simulink model "simulation"  (R2021b)
settings: Solver=VariableStepAuto  StartTime=0.0  StopTime=10.0  RelTol=1e-3
values from neighbouring files (symbols this model uses):
  c0_bar = 1.962390280742725    (= 1.96239028074)    [run_simulation.m]
  DHTABLE = [ pi/2      0         l(1)     q1 ... (first row only)    [compute_vel_obs_gain.m]    (also in dynamic_model_3R_spatial.m = [ pi/2      0      sym('L1') sym('q1'); dynamic_model_simulation.m = [ pi/2      0         l(1)     0; red_obs_gain_computation.m = [ pi/2      0         l(1)     0; run_experiment.m = [ pi/2      0         l(1)     0)
  dq0 = [0.5 -0.5 1]'    [dynamic_model_simulation.m]    (also in run_experiment.m; run_simulation.m = [0., 0., 0.]')
  eta = 1    [compute_vel_obs_gain.m]    (also in dynamic_model_simulation.m; red_obs_gain_computation.m; run_experiment.m; run_simulation.m)
  finite_diff = -1    [run_simulation.m]
  g0 = 9.81    [compute_vel_obs_gain.m]    (also in dynamic_model_3R_spatial.m; dynamic_model_simulation.m; modNE.m = 0; red_obs_gain_computation.m)
  I = zeros(3,3,N)    [compute_vel_obs_gain.m]    (also in dynamic_model_simulation.m; red_obs_gain_computation.m; run_experiment.m; run_simulation.m = zeros(3,3,3))
  K0 = c0bar*(v_max+eta)/(2*lambda_1)    [compute_vel_obs_gain.m]    (also in dynamic_model_simulation.m = 31.0539244645; red_obs_gain_computation.m = 0; run_experiment.m = 103.513081548; run_simulation.m = 62.1078489297)
  K_init = 0.5*dq0'*M*dq0    [run_simulation.m]
  Kd = 3e1    (= 30)    [dynamic_model_simulation.m]    (also in run_experiment.m = 70; run_simulation.m = 50)
  Ko = 5e1    (= 50)    [dynamic_model_simulation.m]    (also in run_experiment.m; run_simulation.m = 10)
  Kp = 3e2    (= 300)    [dynamic_model_simulation.m]    (also in run_experiment.m = 70; run_simulation.m = 100)
  lambda_1 = min(min_first,min_third)/2    [compute_vel_obs_gain.m]    (also in dynamic_model_simulation.m = 0.0947894822263; red_obs_gain_computation.m = min_eig/2; run_experiment.m = 0.0473947411131; run_simulation.m = 0.0473947411131)
  m = [15 10 5]'    [compute_vel_obs_gain.m]    (also in dynamic_model_simulation.m; red_obs_gain_computation.m; run_experiment.m; run_simulation.m = [m1 m2 m3]')
  p_f = [0.,0.8,0.5]    [run_simulation.m]
  p_i = [0.8, 0., 0.5]    [run_simulation.m]
  q0 = inverse_kinematics(p_init,l,soln_type)    [dynamic_model_simulation.m]    (also in run_experiment.m; run_simulation.m = inv_kin(p_i))
  rc = zeros(3,1,3)    [run_simulation.m]
  Timeinterval = [7,9]    [run_simulation.m]
  Timepoints = [0 3 5 7 10]    [run_simulation.m]
  vbar = 2*eta+1    (= 3)    [dynamic_model_simulation.m]    (also in run_simulation.m = 2)
  Velocities = [dq0(1) 2 1 0 -2;dq0(2) 0 2 0 -2;dq0(3) 2 2 0 0]    [run_simulation.m]
  Waypoints = [q0(1) pi/2 pi/4 0 -pi/2; q0(2) pi/4 pi/2 3*pi/4 pi/2; q0(3) pi/2 pi pi/2 -pi/2]    [run_simulation.m]
  x0 = [pi/4,pi/4,1,1,1]'    [compute_vel_obs_gain.m]    (also in dynamic_model_simulation.m = [q0; dq0]; find_c0.m; run_experiment.m = [q0; dq0]; run_simulation.m = [q0;dq0])
  z0 = [0 0 1]'    [dynamic_model_3R_spatial.m]    (also in dynamic_model_simulation.m = x2hat0 - K0*q0; run_experiment.m = x2hat0 - K0*q0; run_simulation.m = x2hat0-K0*q0)
undefined symbols (not defined in the file or in its folder): eul2tform, trvec2tform
libraries: robotcorelib x5, simulink x2, robotmaniplib x1
settings Model: Creator=lyuk  LastModifiedBy=lyuk

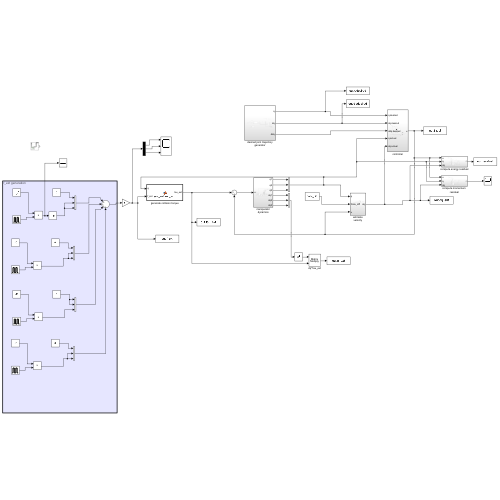
[thumbnail: Simulink's stored preview of the top-level diagram]
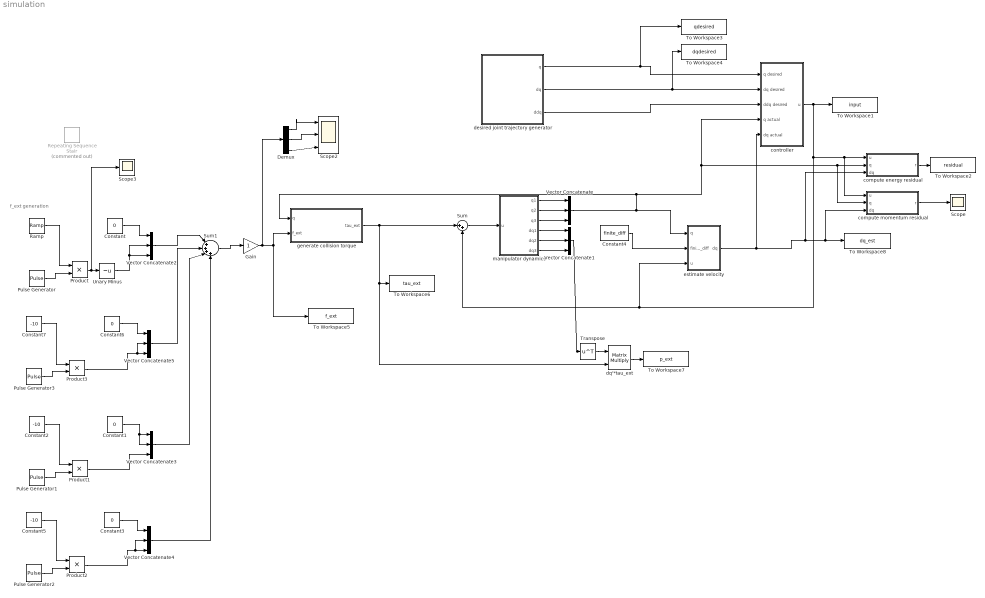
== system simulation ==
  note: f_ext generation
  Constant{,1,3,6} (4 alike) : Constant  Value=0
  Constant2 : Constant  Value=-10
  Constant4 : Constant  Value=finite_diff
  Constant5 : Constant  Value=-10
  Constant7 : Constant  Value=-10
  Demux : Demux  Outputs=3
  Gain : Gain
  Product{,1..3} (4 alike) : Product
  Pulse Generator : DiscretePulseGenerator  PulseType=Time based  Period=10  PulseWidth=20  PhaseDelay=1
  Pulse Generator1 : DiscretePulseGenerator  PulseType=Time based  Period=10  PulseWidth=5  PhaseDelay=7.5
  Pulse Generator2 : DiscretePulseGenerator  PulseType=Time based  Period=10  PulseWidth=5  PhaseDelay=8.5
  Pulse Generator3 : DiscretePulseGenerator  PulseType=Time based  Period=10  PulseWidth=5  PhaseDelay=5
  Ramp : simulink/Sources/Ramp  slope=8  start=1  InitialOutput=0
  Repeating Sequence Stair : simulink/Sources/Repeating Sequence Stair  Commented=on  OutValues=[3 5 15].'  tsamp=-1  OutMin=[]  OutMax=[]  OutDataTypeStr=double  OutputDataTypeScalingMode=double  OutDataType=fixdt(0,8)  ConRadixGroup=Best Precision: Vector-wise  OutScaling=2^-12
  Scope : Scope
  Scope2 : Scope  NumInputPorts=3
  Scope3 : Scope
  Sum : Sum  Inputs=|++
  Sum1 : Sum  Inputs=|++++
  To Workspace1 : ToWorkspace  VariableName=input  SampleTime=-1
  To Workspace2 : ToWorkspace  VariableName=residual  SampleTime=-1
      settings: Save2DSignal=2-D array (concatenate along first dimension)
  To Workspace3 : ToWorkspace  VariableName=qdesired  SampleTime=-1
  To Workspace4 : ToWorkspace  VariableName=dqdesired  SampleTime=-1
  To Workspace5 : ToWorkspace  VariableName=f_ext  SampleTime=-1
  To Workspace6 : ToWorkspace  VariableName=tau_ext  SampleTime=-1
  To Workspace7 : ToWorkspace  VariableName=p_ext  SampleTime=-1
      settings: Save2DSignal=2-D array (concatenate along first dimension)
  To Workspace8 : ToWorkspace  VariableName=dq_est  SampleTime=-1
  Transpose : Math  Operator=transpose  SaturateOnIntegerOverflow=on
  Unary Minus : UnaryMinus
  Vector Concatenate{,1..5} (6 alike) : Concatenate  NumInputs=3  Mode=Multidimensional array
  compute energy residual : Subsystem
  compute momentum residual : Subsystem
  controller : Subsystem
  desired joint trajectory generator : Subsystem
  dq'*tau_ext : Product  Multiplication=Matrix(*)
  estimate velocity : Subsystem
  generate collision torque : MATLAB Function  TreatAsAtomicUnit=on
  manipulator dynamics : Subsystem
  wires:
  manipulator dynamics/2(q2) -> Vector Concatenate/2
  manipulator dynamics/3(q3) -> Vector Concatenate/3
  manipulator dynamics/1(q1) -> Vector Concatenate/1
  manipulator dynamics/4(dq1) -> Vector Concatenate1/1
  manipulator dynamics/5(dq2) -> Vector Concatenate1/2
  manipulator dynamics/6(dq3) -> Vector Concatenate1/3
  Vector Concatenate1/1 -> Transpose/1
  controller/1(u) -> To Workspace1/1, compute momentum residual/1(u), compute energy residual/1(u), estimate velocity/3(u), Sum/2
  compute energy residual/1(r) -> To Workspace2/1
  generate collision torque/1(tau_ext) -> To Workspace6/1, dq'*tau_ext/2, Sum/1
  Sum/1 -> manipulator dynamics/1(u)
  Transpose/1 -> dq'*tau_ext/1
  dq'*tau_ext/1 -> To Workspace7/1
  Product/1 -> Scope3/1, Unary Minus/1
  Pulse Generator/1 -> Product/2
  Ramp/1 -> Product/1
  Vector Concatenate/1 -> estimate velocity/1(q), compute momentum residual/2(q), compute energy residual/2(q), controller/4(q actual), generate collision torque/1(q)
  Unary Minus/1 -> Vector Concatenate2/2, Vector Concatenate2/3
  Constant/1 -> Vector Concatenate2/1
  Gain/1 -> Demux/1, To Workspace5/1, generate collision torque/2(f_ext)
  estimate velocity/1(dq) -> controller/5(dq actual), compute energy residual/3(dq), compute momentum residual/3(dq), To Workspace8/1
  Constant4/1 -> estimate velocity/2(finite_diff)
  compute momentum residual/1(r) -> Scope/1
  desired joint trajectory generator/1(q) -> To Workspace3/1, controller/1(q desired)
  desired joint trajectory generator/2(dq) -> To Workspace4/1, controller/2(dq desired)
  desired joint trajectory generator/3(ddq) -> controller/3(ddq desired)
  Constant1/1 -> Vector Concatenate3/2, Vector Concatenate3/1
  Product1/1 -> Vector Concatenate3/3
  Constant2/1 -> Product1/1
  Pulse Generator1/1 -> Product1/2
  Sum1/1 -> Gain/1
  Vector Concatenate2/1 -> Sum1/1
  Pulse Generator2/1 -> Product2/2
  Constant5/1 -> Product2/1
  Product2/1 -> Vector Concatenate4/2, Vector Concatenate4/3
  Constant3/1 -> Vector Concatenate4/1
  Pulse Generator3/1 -> Product3/2
  Constant7/1 -> Product3/1
  Product3/1 -> Vector Concatenate5/2, Vector Concatenate5/3
  Constant6/1 -> Vector Concatenate5/1
  Vector Concatenate5/1 -> Sum1/2
  Vector Concatenate3/1 -> Sum1/3
  Vector Concatenate4/1 -> Sum1/4
  Demux/1 -> Scope2/1
  Demux/2 -> Scope2/2
  Demux/3 -> Scope2/3

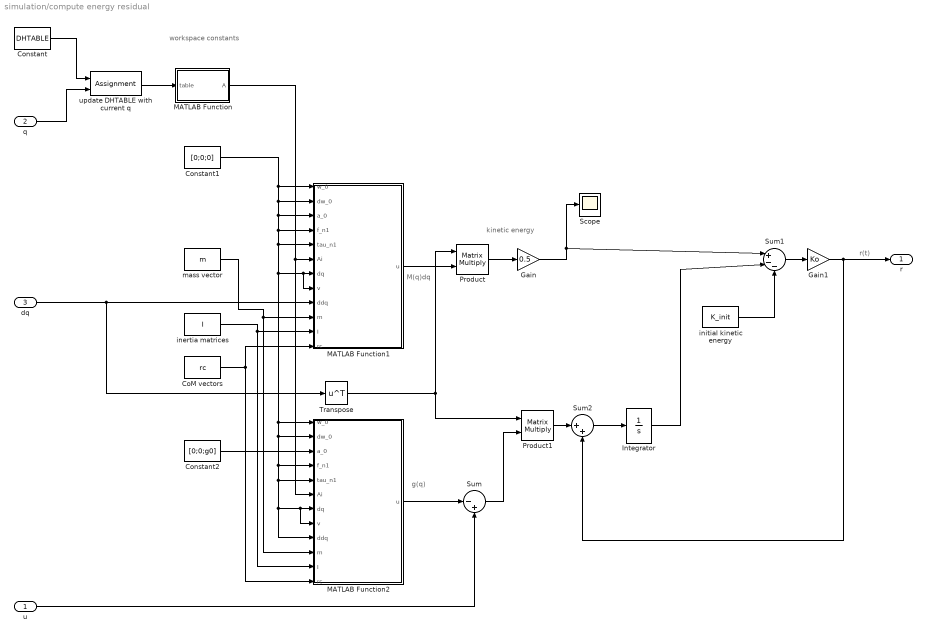
== system simulation/compute energy residual ==
  note: r(t)
  note: g(q)
  note: kinetic energy
  note: M(q)dq
  note: workspace constants
  u : Inport
  q : Inport  Port=2
  dq : Inport  Port=3
  CoM vectors : Constant  Value=rc  VectorParams1D=off
  Constant : Constant  Value=DHTABLE  VectorParams1D=off
  Constant1 : Constant  Value=[0;0;0]  VectorParams1D=off
  Constant2 : Constant  Value=[0;0;g0]  VectorParams1D=off
  Gain : Gain  Gain=0.5
  Gain1 : Gain  Gain=Ko
  Integrator : Integrator
  MATLAB Function : MATLAB Function  TreatAsAtomicUnit=on
  MATLAB Function1 : MATLAB Function  TreatAsAtomicUnit=on
  MATLAB Function2 : MATLAB Function  TreatAsAtomicUnit=on
  Product : Product  Multiplication=Matrix(*)
  Product1 : Product  Multiplication=Matrix(*)
  Scope : Scope
  Sum : Sum  Inputs=|-+
  Sum1 : Sum  Inputs=|+--
  Sum2 : Sum  Inputs=|++
  Transpose : Math  Operator=transpose  SaturateOnIntegerOverflow=on
  inertia matrices : Constant  Value=I  VectorParams1D=off
  initial kinetic energy : Constant  Value=K_init  VectorParams1D=off
  mass vector : Constant  Value=m  VectorParams1D=off
  update DHTABLE with current q : Assignment  NumberOfDimensions=2  DiagnosticForDimensions=Warning  IndexOptions=Assign all,Index vector (dialog)  Indices=1,[4]  OutputSizes=1,1
  r : Outport
  wires:
  mass vector/1 -> MATLAB Function1/10(m), MATLAB Function2/10(m)
  inertia matrices/1 -> MATLAB Function1/11(I), MATLAB Function2/11(I)
  Constant1/1 -> MATLAB Function2/9(ddq), MATLAB Function2/8(v), MATLAB Function2/7(dq), MATLAB Function2/5(tau_n1), MATLAB Function2/4(f_n1), MATLAB Function2/2(dw_0), MATLAB Function2/1(w_0), MATLAB Function1/8(v), MATLAB Function1/7(dq), MATLAB Function1/5(tau_n1), MATLAB Function1/4(f_n1), MATLAB Function1/3(a_0), MATLAB Function1/2(dw_0), MATLAB Function1/1(w_0)
  CoM vectors/1 -> MATLAB Function1/12(rc), MATLAB Function2/12(rc)
  update DHTABLE with current q/1 -> MATLAB Function/1(table)
  Constant/1 -> update DHTABLE with current q/1
  MATLAB Function/1(A) -> MATLAB Function2/6(Ai), MATLAB Function1/6(Ai)
  q/1 -> update DHTABLE with current q/2
  dq/1 -> Transpose/1, MATLAB Function1/9(ddq)
  MATLAB Function1/1(u) -> Product/2
  Transpose/1 -> Product/1, Product1/1
  Product/1 -> Gain/1
  Constant2/1 -> MATLAB Function2/3(a_0)
  Gain1/1 -> Sum2/2, r/1
  u/1 -> Sum/2
  Sum/1 -> Product1/2
  Gain/1 -> Scope/1, Sum1/1
  Integrator/1 -> Sum1/2
  Sum1/1 -> Gain1/1
  Product1/1 -> Sum2/1
  Sum2/1 -> Integrator/1
  MATLAB Function2/1(u) -> Sum/1
  initial kinetic energy/1 -> Sum1/3

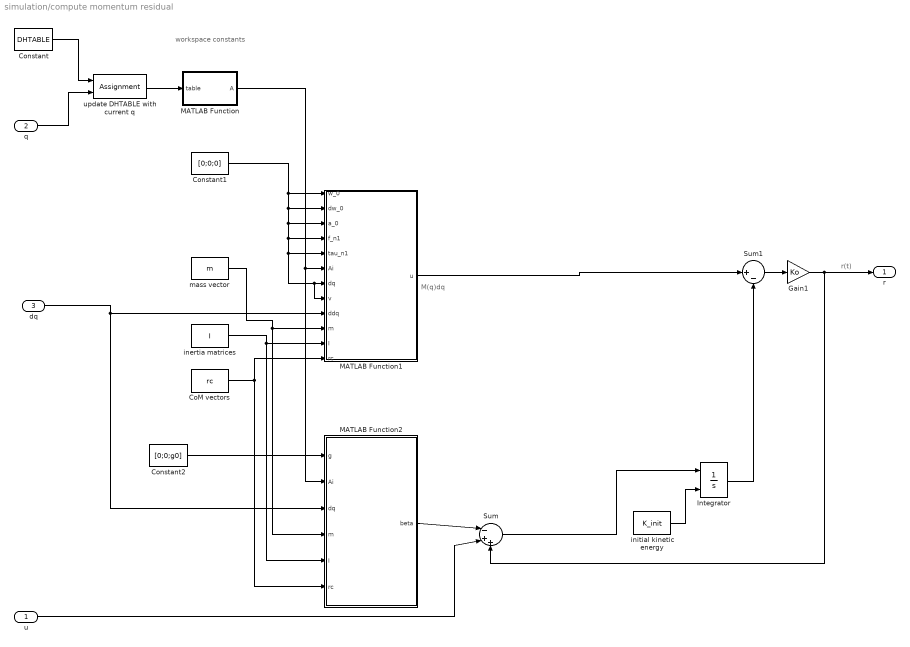
== system simulation/compute momentum residual ==
  note: workspace constants
  note: M(q)dq
  note: r(t)
  u : Inport
  q : Inport  Port=2
  dq : Inport  Port=3
  CoM vectors : Constant  Value=rc  VectorParams1D=off
  Constant : Constant  Value=DHTABLE  VectorParams1D=off
  Constant1 : Constant  Value=[0;0;0]  VectorParams1D=off
  Constant2 : Constant  Value=[0;0;g0]  VectorParams1D=off
  Gain1 : Gain  Gain=Ko
  Integrator : Integrator  InitialConditionSource=external
  MATLAB Function : MATLAB Function  TreatAsAtomicUnit=on
  MATLAB Function1 : MATLAB Function  TreatAsAtomicUnit=on
  MATLAB Function2 : MATLAB Function  TreatAsAtomicUnit=on
  Sum : Sum  Inputs=|-++
  Sum1 : Sum  Inputs=|+-
  inertia matrices : Constant  Value=I  VectorParams1D=off
  initial kinetic energy : Constant  Value=K_init  VectorParams1D=off
  mass vector : Constant  Value=m  VectorParams1D=off
  update DHTABLE with current q : Assignment  NumberOfDimensions=2  DiagnosticForDimensions=Warning  IndexOptions=Assign all,Index vector (dialog)  Indices=1,[4]  OutputSizes=1,1
  r : Outport
  wires:
  Sum/1 -> Integrator/1
  initial kinetic energy/1 -> Integrator/2
  Sum1/1 -> Gain1/1
  Integrator/1 -> Sum1/2
  u/1 -> Sum/2
  MATLAB Function2/1(beta) -> Sum/1
  Gain1/1 -> Sum/3, r/1
  Constant2/1 -> MATLAB Function2/1(g)
  MATLAB Function1/1(u) -> Sum1/1
  dq/1 -> MATLAB Function1/9(ddq), MATLAB Function2/3(dq)
  q/1 -> update DHTABLE with current q/2
  MATLAB Function/1(A) -> MATLAB Function1/6(Ai), MATLAB Function2/2(Ai)
  Constant/1 -> update DHTABLE with current q/1
  update DHTABLE with current q/1 -> MATLAB Function/1(table)
  CoM vectors/1 -> MATLAB Function2/6(rc), MATLAB Function1/12(rc)
  Constant1/1 -> MATLAB Function1/1(w_0), MATLAB Function1/2(dw_0), MATLAB Function1/3(a_0), MATLAB Function1/4(f_n1), MATLAB Function1/5(tau_n1), MATLAB Function1/7(dq), MATLAB Function1/8(v)
  inertia matrices/1 -> MATLAB Function2/5(I), MATLAB Function1/11(I)
  mass vector/1 -> MATLAB Function2/4(m), MATLAB Function1/10(m)

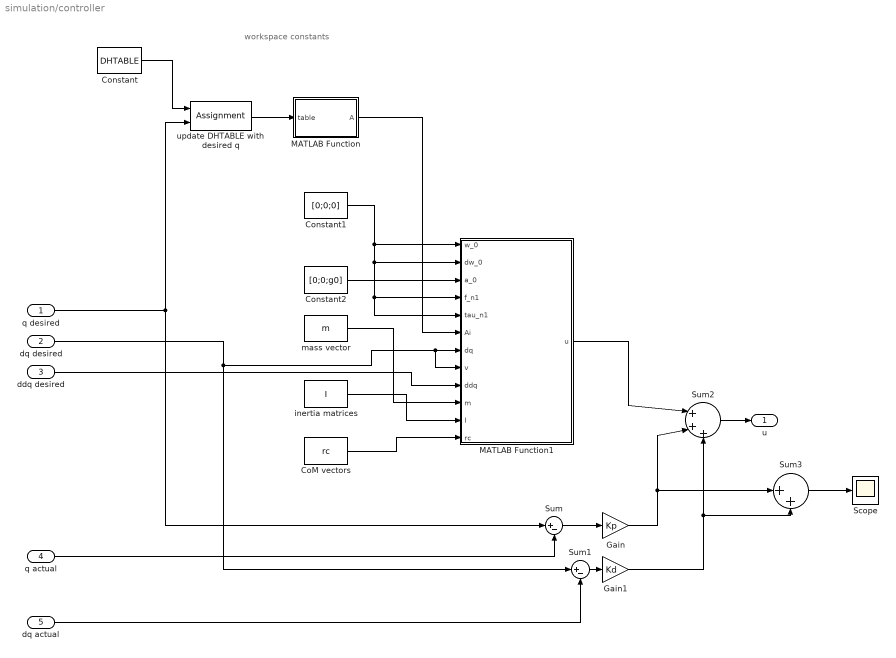
== system simulation/controller ==
  note: workspace constants
  q desired : Inport
  dq desired : Inport  Port=2
  ddq desired : Inport  Port=3
  q actual : Inport  Port=4
  dq actual : Inport  Port=5
  CoM vectors : Constant  Value=rc  VectorParams1D=off
  Constant : Constant  Value=DHTABLE  VectorParams1D=off
  Constant1 : Constant  Value=[0;0;0]  VectorParams1D=off
  Constant2 : Constant  Value=[0;0;g0]  VectorParams1D=off
  Gain : Gain  Gain=Kp
  Gain1 : Gain  Gain=Kd
  MATLAB Function : MATLAB Function  TreatAsAtomicUnit=on
  MATLAB Function1 : MATLAB Function  TreatAsAtomicUnit=on
  Scope : Scope
  Sum : Sum  Inputs=|+-
  Sum1 : Sum  Inputs=|+-
  Sum2 : Sum  Inputs=|+++
  Sum3 : Sum  Inputs=|++
  inertia matrices : Constant  Value=I  VectorParams1D=off
  mass vector : Constant  Value=m  VectorParams1D=off
  update DHTABLE with desired q : Assignment  NumberOfDimensions=2  DiagnosticForDimensions=Warning  IndexOptions=Assign all,Index vector (dialog)  Indices=1,[4]  OutputSizes=1,1
  u : Outport
  wires:
  Gain1/1 -> Sum3/2, Sum2/3
  update DHTABLE with desired q/1 -> MATLAB Function/1(table)
  Gain/1 -> Sum2/2, Sum3/1
  Constant/1 -> update DHTABLE with desired q/1
  Constant1/1 -> MATLAB Function1/2(dw_0), MATLAB Function1/5(tau_n1), MATLAB Function1/4(f_n1), MATLAB Function1/1(w_0)
  inertia matrices/1 -> MATLAB Function1/11(I)
  CoM vectors/1 -> MATLAB Function1/12(rc)
  Constant2/1 -> MATLAB Function1/3(a_0)
  mass vector/1 -> MATLAB Function1/10(m)
  MATLAB Function/1(A) -> MATLAB Function1/6(Ai)
  Sum1/1 -> Gain1/1
  q desired/1 -> Sum/1, update DHTABLE with desired q/2
  dq desired/1 -> MATLAB Function1/8(v), MATLAB Function1/7(dq), Sum1/1
  ddq desired/1 -> MATLAB Function1/9(ddq)
  dq actual/1 -> Sum1/2
  Sum/1 -> Gain/1
  q actual/1 -> Sum/2
  Sum3/1 -> Scope/1
  Sum2/1 -> u/1
  MATLAB Function1/1(u) -> Sum2/1

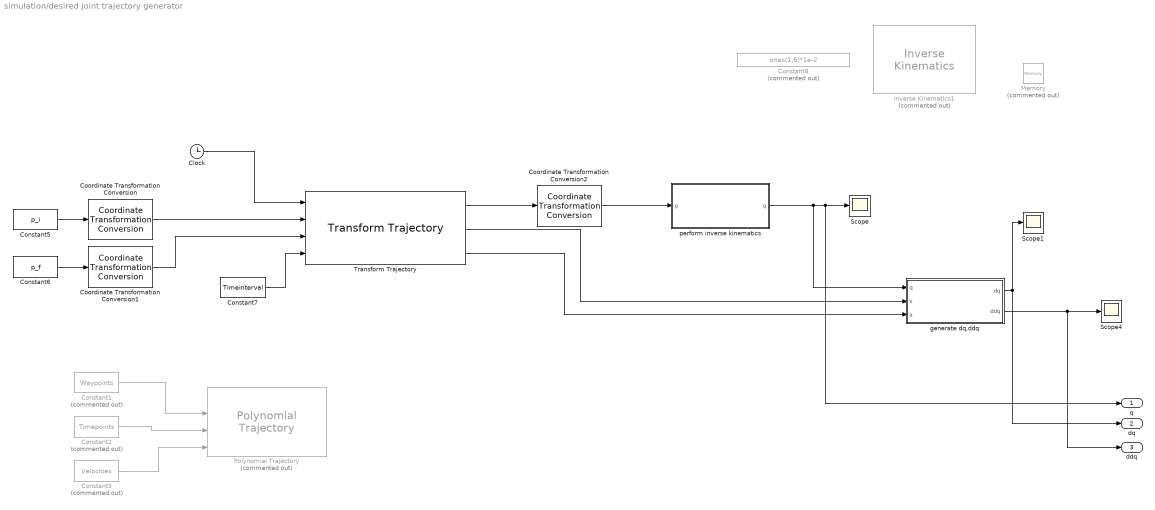
== system simulation/desired joint trajectory generator ==
  Clock : Clock
  Constant1 : Constant  Commented=on  Value=Waypoints
  Constant2 : Constant  Commented=on  Value=Timepoints
  Constant3 : Constant  Commented=on  Value=Velocities
  Constant5 : Constant  Value=p_i
  Constant6 : Constant  Value=p_f
  Constant7 : Constant  Value=Timeinterval
  Constant8 : Constant  Commented=on  Value=ones(1,6)*1e-2
  Coordinate Transformation Conversion : robotcorelib/Coordinate Transformation Conversion  InputRepresentation=Translation Vector  InputEulerSequence=ZYX  ShowTrVecInputPort=on  OutputRepresentation=Homogeneous Transformation  OutputEulerSequence=ZYX  ShowTrVecOutputPort=on  SimulateUsing=Interpreted execution
      settings: SourceProductBaseCode=NV,RO,RR,UV
  Coordinate Transformation Conversion1 : robotcorelib/Coordinate Transformation Conversion  InputRepresentation=Translation Vector  InputEulerSequence=ZYX  ShowTrVecInputPort=on  OutputRepresentation=Homogeneous Transformation  OutputEulerSequence=ZYX  ShowTrVecOutputPort=on  SimulateUsing=Interpreted execution
      settings: SourceProductBaseCode=NV,RO,RR,UV
  Coordinate Transformation Conversion2 : robotcorelib/Coordinate Transformation Conversion  InputRepresentation=Homogeneous Transformation  InputEulerSequence=ZYX  ShowTrVecInputPort=on  OutputRepresentation=Translation Vector  OutputEulerSequence=ZYX  ShowTrVecOutputPort=on  SimulateUsing=Interpreted execution
      settings: SourceProductBaseCode=NV,RO,RR,UV
  Inverse Kinematics1 : robotmaniplib/Inverse Kinematics  Commented=on  RigidBodyTree=robot  EndEffector=body3  ShowInfo=on  SolverName=BFGS Gradient Projection  EnforceJointLimits=on  MaxIterations=1500  MaxTime=10  GradientTolerance=1e-7  SolutionTolerance=1e-6  StepTolerance=1e-14  ErrorChangeTolerance=1e-12  UseErrorDamping=on  DampingBias=0.0025  SimulateUsing=Interpreted execution
  Memory : Memory  Commented=on  InitialCondition=q0  InheritSampleTime=on
  Polynomial Trajectory : robotcorelib/Polynomial Trajectory  Commented=on  WaypointSource=External  Waypoints=[q0(1) pi/2 pi; q0(2) pi/4 pi/2; q0(3) pi/2 0]  TimePoints=[0 5 10 ]  TimeInterval=[ 1, 4 ]  Method=Cubic Polynomial  ParameterSource=External  VelocityBoundaryCondition=[dq0(1) zeros(1,2);dq0(2) zeros(1,2);dq0(3) zeros(1,2)]  AccelerationBoundaryCondition=zeros( 2, 5 )  SimulateUsing=Interpreted execution
  Scope : Scope
  Scope1 : Scope
  Scope4 : Scope
  Transform Trajectory : robotcorelib/Transform Trajectory  WaypointSource=External  T0=trvec2tform( [ 1, 10, -1 ] )  TF=eul2tform( [ 0, pi, pi / 2 ] )  TimeInterval=[ 2, 3 ]  CustomTimeScaling=off  ParameterSource=Internal  TSTime=2:0.1:3  TimeScaling=[ 0:0.1:1; ones( 1, 11 ); zeros( 1, 11 ) ]  SimulateUsing=Interpreted execution
      settings: SourceProductBaseCode=NV,RO,RR,UV
  generate dq,ddq : MATLAB Function  TreatAsAtomicUnit=on
  perform inverse kinematics : MATLAB Function  TreatAsAtomicUnit=on
  q : Outport
  dq : Outport  Port=2
  ddq : Outport  Port=3
  wires:
  perform inverse kinematics/1(q) -> q/1, Scope/1, generate dq,ddq/1(q)
  Constant2/1 -> Polynomial Trajectory/3
  Constant3/1 -> Polynomial Trajectory/4
  Clock/1 -> Transform Trajectory/1
  Constant1/1 -> Polynomial Trajectory/2
  Constant7/1 -> Transform Trajectory/4
  Transform Trajectory/2 -> generate dq,ddq/2(v)
  Transform Trajectory/3 -> generate dq,ddq/3(a)
  generate dq,ddq/1(dq) -> dq/1, Scope1/1
  generate dq,ddq/2(ddq) -> Scope4/1, ddq/1
  Constant5/1 -> Coordinate Transformation Conversion/1
  Coordinate Transformation Conversion/1 -> Transform Trajectory/2
  Constant6/1 -> Coordinate Transformation Conversion1/1
  Coordinate Transformation Conversion1/1 -> Transform Trajectory/3
  Coordinate Transformation Conversion2/1 -> perform inverse kinematics/1(p)
  Transform Trajectory/1 -> Coordinate Transformation Conversion2/1

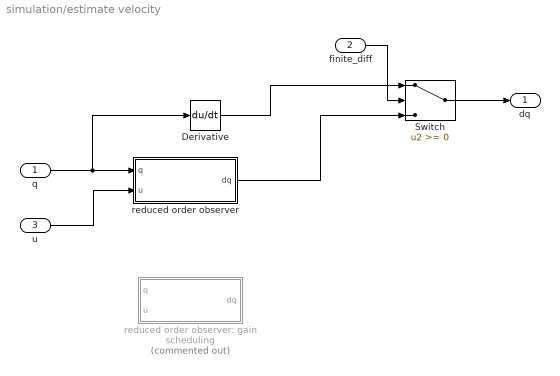
== system simulation/estimate velocity ==
  q : Inport
  finite_diff : Inport  Port=2
  u : Inport  Port=3
  Derivative : Derivative
  Switch : Switch
  reduced order observer : Subsystem
  reduced order observer: gain scheduling : Subsystem  Commented=on
  dq : Outport
  wires:
  q/1 -> Derivative/1, reduced order observer/1(q)
  reduced order observer/1(dq) -> Switch/3
  Switch/1 -> dq/1
  Derivative/1 -> Switch/1
  finite_diff/1 -> Switch/2
  u/1 -> reduced order observer/2(u)

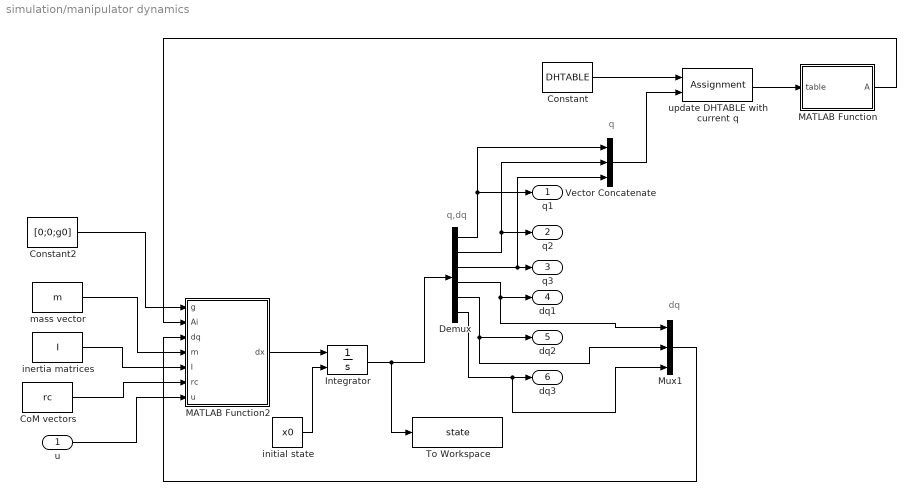
== system simulation/manipulator dynamics ==
  note: q
  note: q,dq
  note: dq
  u : Inport
  CoM vectors : Constant  Value=rc  VectorParams1D=off
  Constant : Constant  Value=DHTABLE  VectorParams1D=off
  Constant2 : Constant  Value=[0;0;g0]  VectorParams1D=off
  Demux : Demux  Outputs=6
  Integrator : Integrator  InitialConditionSource=external  InitialCondition=[q0;dq0]
  MATLAB Function : MATLAB Function  TreatAsAtomicUnit=on
  MATLAB Function2 : MATLAB Function  TreatAsAtomicUnit=on
  Mux1 : Mux  Inputs=3
  To Workspace : ToWorkspace  VariableName=state  SampleTime=-1
  Vector Concatenate : Concatenate  NumInputs=3  Mode=Multidimensional array
  inertia matrices : Constant  Value=I  VectorParams1D=off
  initial state : Constant  Value=x0  VectorParams1D=off
  mass vector : Constant  Value=m  VectorParams1D=off
  update DHTABLE with current q : Assignment  NumberOfDimensions=2  DiagnosticForDimensions=Warning  IndexOptions=Assign all,Index vector (dialog)  Indices=1,[4]  OutputSizes=1,1
  q1 : Outport
  q2 : Outport  Port=2
  q3 : Outport  Port=3
  dq1 : Outport  Port=4
  dq2 : Outport  Port=5
  dq3 : Outport  Port=6
  wires:
  Demux/1 -> q1/1, Vector Concatenate/1
  Integrator/1 -> To Workspace/1, Demux/1
  Demux/6 -> Mux1/3, dq3/1
  Demux/4 -> Mux1/1, dq1/1
  u/1 -> MATLAB Function2/7(u)
  Demux/2 -> Vector Concatenate/2, q2/1
  MATLAB Function2/1(dx) -> Integrator/1
  Demux/3 -> Vector Concatenate/3, q3/1
  Demux/5 -> dq2/1, Mux1/2
  update DHTABLE with current q/1 -> MATLAB Function/1(table)
  mass vector/1 -> MATLAB Function2/4(m)
  inertia matrices/1 -> MATLAB Function2/5(I)
  CoM vectors/1 -> MATLAB Function2/6(rc)
  Mux1/1 -> MATLAB Function2/3(dq)
  Vector Concatenate/1 -> update DHTABLE with current q/2
  Constant/1 -> update DHTABLE with current q/1
  MATLAB Function/1(A) -> MATLAB Function2/2(Ai)
  Constant2/1 -> MATLAB Function2/1(g)
  initial state/1 -> Integrator/2

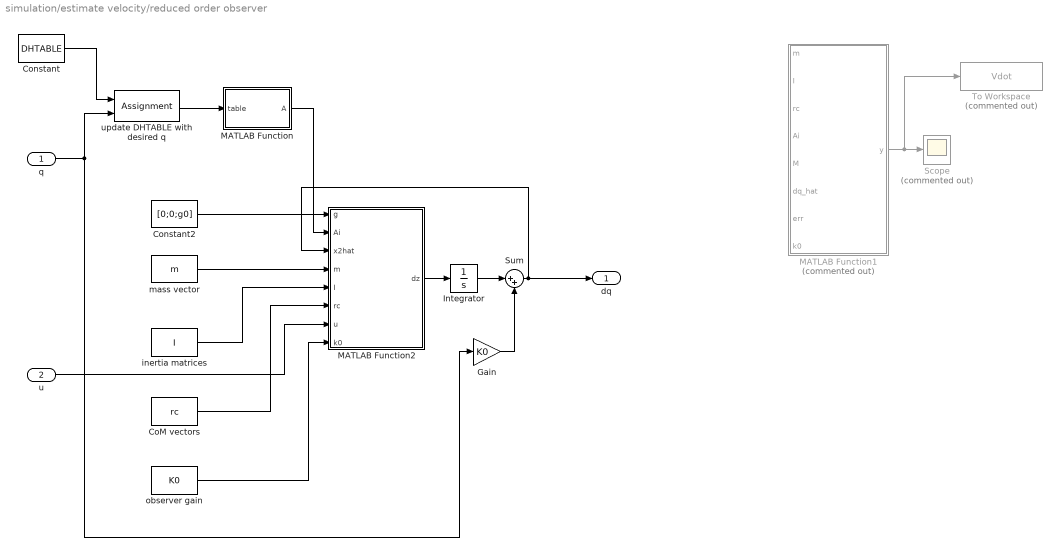
== system simulation/estimate velocity/reduced order observer ==
  q : Inport
  u : Inport  Port=2
  CoM vectors : Constant  Value=rc  VectorParams1D=off
  Constant : Constant  Value=DHTABLE  VectorParams1D=off
  Constant2 : Constant  Value=[0;0;g0]  VectorParams1D=off
  Gain : Gain  Gain=K0
  Integrator : Integrator  InitialCondition=z0
  MATLAB Function : MATLAB Function  TreatAsAtomicUnit=on
  MATLAB Function1 : MATLAB Function  Commented=on  TreatAsAtomicUnit=on
  MATLAB Function2 : MATLAB Function  TreatAsAtomicUnit=on
  Scope : Scope  Commented=on
  Sum : Sum  Inputs=|++
  To Workspace : ToWorkspace  Commented=on  VariableName=Vdot  SampleTime=-1
  inertia matrices : Constant  Value=I  VectorParams1D=off
  mass vector : Constant  Value=m  VectorParams1D=off
  observer gain : Constant  Value=K0  VectorParams1D=off
  update DHTABLE with desired q : Assignment  NumberOfDimensions=2  DiagnosticForDimensions=Warning  IndexOptions=Assign all,Index vector (dialog)  Indices=1,[4]  OutputSizes=1,1
  dq : Outport
  wires:
  CoM vectors/1 -> MATLAB Function2/6(rc)
  inertia matrices/1 -> MATLAB Function2/5(I)
  mass vector/1 -> MATLAB Function2/4(m)
  Constant2/1 -> MATLAB Function2/1(g)
  update DHTABLE with desired q/1 -> MATLAB Function/1(table)
  Constant/1 -> update DHTABLE with desired q/1
  q/1 -> update DHTABLE with desired q/2, Gain/1
  MATLAB Function/1(A) -> MATLAB Function2/2(Ai)
  observer gain/1 -> MATLAB Function2/8(k0)
  u/1 -> MATLAB Function2/7(u)
  MATLAB Function2/1(dz) -> Integrator/1
  Integrator/1 -> Sum/1
  Gain/1 -> Sum/2
  Sum/1 -> dq/1, MATLAB Function2/3(x2hat)
  MATLAB Function1/1(y) -> To Workspace/1, Scope/1

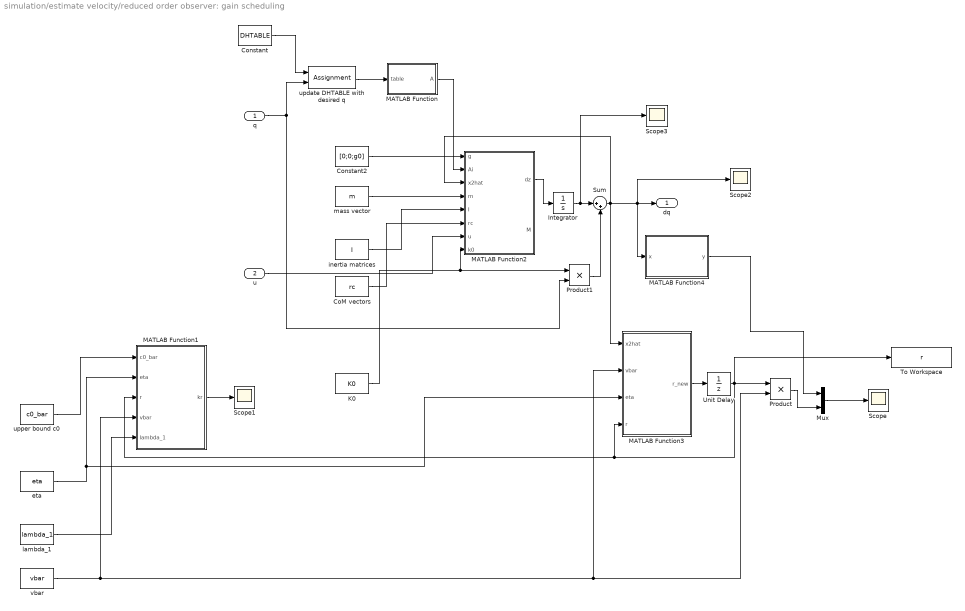
== system simulation/estimate velocity/reduced order observer: gain scheduling ==
  q : Inport
  u : Inport  Port=2
  CoM vectors : Constant  Value=rc  VectorParams1D=off
  Constant : Constant  Value=DHTABLE  VectorParams1D=off
  Constant2 : Constant  Value=[0;0;g0]  VectorParams1D=off
  Integrator : Integrator  InitialCondition=z0
  K0 : Constant  Value=K0  VectorParams1D=off
  MATLAB Function : MATLAB Function  TreatAsAtomicUnit=on
  MATLAB Function1 : MATLAB Function  TreatAsAtomicUnit=on
  MATLAB Function2 : MATLAB Function  TreatAsAtomicUnit=on
  MATLAB Function3 : MATLAB Function  TreatAsAtomicUnit=on
  MATLAB Function4 : MATLAB Function  TreatAsAtomicUnit=on
  Mux : Mux  Inputs=2
  Product : Product
  Product1 : Product
  Scope{,1..3} (4 alike) : Scope
  Sum : Sum  Inputs=|++
  To Workspace : ToWorkspace  VariableName=r  SaveFormat=Structure With Time  SampleTime=-1
  Unit Delay : UnitDelay  InitialCondition=1  SampleTime=-1  HasFrameUpgradeWarning=on
  eta : Constant  Value=eta  VectorParams1D=off
  inertia matrices : Constant  Value=I  VectorParams1D=off
  lambda_1 : Constant  Value=lambda_1  VectorParams1D=off
  mass vector : Constant  Value=m  VectorParams1D=off
  update DHTABLE with desired q : Assignment  NumberOfDimensions=2  DiagnosticForDimensions=Warning  IndexOptions=Assign all,Index vector (dialog)  Indices=1,[4]  OutputSizes=1,1
  upper bound c0 : Constant  Value=c0_bar  VectorParams1D=off
  vbar : Constant  Value=vbar  VectorParams1D=off
  dq : Outport
  wires:
  Sum/1 -> Scope2/1, MATLAB Function4/1(x), dq/1, MATLAB Function3/1(x2hat), MATLAB Function2/3(x2hat)
  Product1/1 -> Sum/2
  Integrator/1 -> Scope3/1, Sum/1
  MATLAB Function2/1(dz) -> Integrator/1
  u/1 -> MATLAB Function2/7(u)
  MATLAB Function/1(A) -> MATLAB Function2/2(Ai)
  q/1 -> Product1/2, update DHTABLE with desired q/2
  Constant/1 -> update DHTABLE with desired q/1
  update DHTABLE with desired q/1 -> MATLAB Function/1(table)
  Constant2/1 -> MATLAB Function2/1(g)
  mass vector/1 -> MATLAB Function2/4(m)
  inertia matrices/1 -> MATLAB Function2/5(I)
  CoM vectors/1 -> MATLAB Function2/6(rc)
  upper bound c0/1 -> MATLAB Function1/1(c0_bar)
  eta/1 -> MATLAB Function3/3(eta), MATLAB Function1/2(eta)
  lambda_1/1 -> MATLAB Function1/5(lambda_1)
  vbar/1 -> MATLAB Function1/4(vbar), Product/2, MATLAB Function3/2(vbar)
  MATLAB Function3/1(r_new) -> Unit Delay/1
  MATLAB Function1/1(kr) -> Scope1/1
  MATLAB Function4/1(y) -> Mux/1
  Product/1 -> Mux/2
  Mux/1 -> Scope/1
  Unit Delay/1 -> MATLAB Function3/4(r), MATLAB Function1/3(r), To Workspace/1, Product/1
  K0/1 -> MATLAB Function2/8(k0), Product1/1

== matlab function simulation/compute momentum residual/MATLAB Function ==
  data: table input; A output
function A = DHMatrix(table)
% inputs:
%  -table: the DH parameters table, a n-vector of vectors composed with 
%  this structure: [alpha a d theta]
% output:
%  -A: cell array with homogeneous relative transformations from RF i-1 to
%   RF i
    nums = size(table);
    
    A = zeros(4,4,nums(1));
    
    for i = 1:nums(1)
        line = table(i, :);
        R = [cos(line(4)) -cos(line(1))*sin(line(4)) sin(line(1))*sin(line(4)) line(2)*cos(line(4));
             sin(line(4)) cos(line(1))*cos(line(4)) -sin(line(1))*cos(line(4)) line(2)*sin(line(4));
             0 sin(line(1)) cos(line(1)) line(3);
             0 0 0 1;];
        A(:,:,i) = R;
    end
   
end

== matlab function simulation/generate collision torque ==
  data: q input size=[3,1]; f_ext input size=[3,1]; tau_ext output
function tau_ext = gen_collision_torq(q, f_ext)

J = [-(sin(q(1))*(4*cos(q(2) + q(3)) + 5*cos(q(2))))/10, -(cos(q(1))*(4*sin(q(2) + q(3)) + 5*sin(q(2))))/10, -(2*sin(q(2) + q(3))*cos(q(1)))/5;
    (cos(q(1))*(4*cos(q(2) + q(3)) + 5*cos(q(2))))/10, -(sin(q(1))*(4*sin(q(2) + q(3)) + 5*sin(q(2))))/10, -(2*sin(q(2) + q(3))*sin(q(1)))/5;
                                            0,             (2*cos(q(2) + q(3)))/5 + cos(q(2))/2,          (2*cos(q(2) + q(3)))/5];
tau_ext = J'*f_ext;
end

== matlab function simulation/compute momentum residual/MATLAB Function1 ==
  data: w_0 input; u output; dw_0 input; a_0 input; f_n1 input; tau_n1 input; Ai input; dq input; v input; ddq input; m input; I input; rc input
function u=mod_newton_euler(w_0,dw_0,a_0,f_n1,tau_n1,Ai,dq,v,ddq,m,I,rc)
% NE algorithm for robot dynamics with revolute joints
% inputs:
% - w_0, dw_0: angular velocity and acceleration of the base
%  - a_0: acceleration of the base (set this to -g to consider gravity)
%  - f_n1,tau_n1: force and torque vectors applied at the end effector, 0 if not in contact with environment
%  - Ai: 4x4xn matrix with the 4x4 DH homogeneous matrices
%  - dq, ddq: joint velocity and acceleration
%  - v: velocity multiplying matrix C(q,dq)
%  - m: n-dimensional array with link masses
%  - I: 3x3xn matrix containing inertia matrices
%  - rc: 3x1xn matrix with CoM vectors of link i expressed in frame i

n=size(Ai,3);

R=zeros(3,3,n);
for i=1:n
    R(:,:,i)=Ai(1:3,1:3,i);
end

w=zeros(3,1,n); 
w(:,:,1)=R(:,:,1)'*(w_0+[0;0;dq(1)]);

wa=zeros(3,1,n);
wa_0=zeros(3,1);
wa(:,:,1)=R(:,:,1)'*(wa_0+[0;0;v(1)]);

dw=zeros(3,1,n); 
dw(:,:,1)=R(:,:,1)'*(dw_0+[0;0;ddq(1)] + dq(1)*cross(wa_0,[0;0;1]));

a=zeros(3,1,n);
a(:,:,1)=R(:,:,1)'*a_0 + cross(dw(:,:,1),R(:,:,1)'*Ai(1:3,4,1)) + cross(w(:,:,1),cross(wa(:,:,1),R(:,:,1)'*Ai(1:3,4,1)));

ac=zeros(3,1,n);
ac(:,:,1)= a(:,:,1) + cross(dw(:,:,1),rc(:,:,1)) + cross(w(:,:,1),cross(wa(:,:,1),rc(:,:,1)));

%forward recursion
for i=2:n
    w(:,:,i)=R(:,:,i)'*(w(:,:,i-1)+[0;0;dq(i)]);
    wa(:,:,i)=R(:,:,i)'*(wa(:,:,i-1)+[0;0;v(i)]);
    dw(:,:,i)=R(:,:,i)'*( dw(:,:,i-1)+[0;0;ddq(i)] + dq(i)*(Smtrx(wa(:,:,i-1))*[0;0;1]));
    a(:,:,i)=R(:,:,i)'*a(:,:,i-1) + cross(dw(:,:,i),R(:,:,i)'*Ai(1:3,4,i)) + cross(w(:,:,i),cross(wa(:,:,i), R(:,:,i)'*Ai(1:3,4,i)));
    ac(:,:,i)= a(:,:,i) + cross(dw(:,:,i),rc(:,:,i)) + cross(w(:,:,i),cross(wa(:,:,i),rc(:,:,i)));
end

%backward recursion
f=zeros(3,1,n);
f(:,:,n)= f_n1 + m(n)*ac(:,:,n);
tau=zeros(3,1,n);
tau(:,:,n)= tau_n1 + cross(f_n1,rc(:,:,n)) - cross(f(:,:,n),R(:,:,n)'*Ai(1:3,4,n) + rc(:,:,n)) + I(:,:,n)*dw(:,:,n) + cross(wa(:,:,n),I(:,:,n)*w(:,:,n));
for i=n-1:-1:1
    f(:,:,i)= R(:,:,i+1)*f(:,:,i+1) + m(i)*ac(:,:,i);
    tau(:,:,i)= R(:,:,i+1)*tau(:,:,i+1) + cross(R(:,:,i+1)*f(:,:,i+1),rc(:,:,i)) - cross(f(:,:,i),R(:,:,i)'*Ai(1:3,4,i) + rc(:,:,i)) + I(:,:,i)*dw(:,:,i) + cross(wa(:,:,i),I(:,:,i)*w(:,:,i));
end

% projection
u=zeros(n,1);
for i=1:n
    u(i)=tau(:,:,i)'*R(3,:,i)';
end

== matlab function simulation/compute momentum residual/MATLAB Function2 ==
  data: g input; beta output; Ai input; dq input; m input; I input; rc input
function beta=get_beta(g,Ai,dq,m,I,rc)
% NE algorithm for robot dynamics with revolute joints
% inputs:
% - w_0, dw_0: angular velocity and acceleration of the base
%  - a_0: acceleration of the base (set this to -g to consider gravity)
%  - f_n1,tau_n1: force and torque vectors applied at the end effector, 0 if not in contact with environment
%  - Ai: 4x4xn matrix with the 4x4 DH homogeneous matrices
%  - dq, ddq: joint velocity and acceleration
%  - v: velocity multiplying matrix C(q,dq)
%  - m: n-dimensional array with link masses
%  - I: 3x3xn matrix containing inertia matrices
%  - rc: 3x1xn matrix with CoM vectors of link i expressed in frame i

C=zeros(3,3);
C(:,1)=mod_newton_euler([0;0;0],[0;0;0],[0;0;0],[0;0;0],[0;0;0],Ai,dq,[1;0;0],[0;0;0],m,I,rc);
C(:,2)=mod_newton_euler([0;0;0],[0;0;0],[0;0;0],[0;0;0],[0;0;0],Ai,dq,[0;1;0],[0;0;0],m,I,rc);
C(:,3)=mod_newton_euler([0;0;0],[0;0;0],[0;0;0],[0;0;0],[0;0;0],Ai,dq,[0;0;1],[0;0;0],m,I,rc);
G=mod_newton_euler([0;0;0],[0;0;0],g,[0;0;0],[0;0;0],Ai,[0;0;0],[0;0;0],[0;0;0],m,I,rc);

beta = G-C'*dq;

== matlab function simulation/estimate velocity/reduced order observer/MATLAB Function2 ==
  data: g input; Ai input; x2hat input; m input; I input; rc input; dz output; u input; k0 input
function dz= obs_dynamics(g,Ai,x2hat,m,I,rc,u,k0)
% return the continuous time dynamics given state  and input

Cg = mod_newton_euler(zeros(3,1),zeros(3,1),g,zeros(3,1),zeros(3,1), ...
    Ai,x2hat,x2hat,zeros(3,1),m,I,rc);

M = zeros(3,3);
M(:,1) = mod_newton_euler(zeros(3,1),zeros(3,1),zeros(3,1),zeros(3,1),zeros(3,1), ...
        Ai,zeros(3,1),zeros(3,1),[1;0;0],m,I,rc);
M(:,2) = mod_newton_euler(zeros(3,1),zeros(3,1),zeros(3,1),zeros(3,1),zeros(3,1), ...
        Ai,zeros(3,1),zeros(3,1),[0;1;0],m,I,rc);
M(:,3) = mod_newton_euler(zeros(3,1),zeros(3,1),zeros(3,1),zeros(3,1),zeros(3,1), ...
        Ai,zeros(3,1),zeros(3,1),[0;0;1],m,I,rc);

dz = inv(M)*(-Cg+u)-k0*x2hat;
end

== matlab function simulation/estimate velocity/reduced order observer/MATLAB Function ==
  data: table input; A output
function A = DHMatrix(table)
% inputs:
%  -table: the DH parameters table, a n-vector of vectors composed with 
%  this structure: [alpha a d theta]
% output:
%  -A: cell array with homogeneous relative transformations from RF i-1 to
%   RF i
    nums = size(table);
    
    A = zeros(4,4,nums(1));
    
    for i = 1:nums(1)
        line = table(i, :);
        R = [cos(line(4)) -cos(line(1))*sin(line(4)) sin(line(1))*sin(line(4)) line(2)*cos(line(4));
             sin(line(4)) cos(line(1))*cos(line(4)) -sin(line(1))*cos(line(4)) line(2)*sin(line(4));
             0 sin(line(1)) cos(line(1)) line(3);
             0 0 0 1;];
        A(:,:,i) = R;
    end
   
end

== matlab function simulation/estimate velocity/reduced order observer/MATLAB Function1 ==
  data: m input; I input; rc input; Ai input; M input; dq_hat input; err input; y output; k0 input
function y = Vdot(m,I,rc,Ai,M,dq_hat,err,k0)

C = mod_newton_euler(zeros(3,1),zeros(3,1),zeros(3,1),zeros(3,1),zeros(3,1), ...
    Ai,dq_hat,err,zeros(3,1),m,I,rc);

y = -err'*C-err'*M*k0*err;

== matlab function simulation/controller/MATLAB Function1 ==
  data: w_0 input; u output; dw_0 input; a_0 input; f_n1 input; tau_n1 input; Ai input; dq input; v input; ddq input; m input; I input; rc input
function u=mod_newton_euler(w_0,dw_0,a_0,f_n1,tau_n1,Ai,dq,v,ddq,m,I,rc)
% NE algorithm for robot dynamics with revolute joints
% inputs:
% - w_0, dw_0: angular velocity and acceleration of the base
%  - a_0: acceleration of the base (set this to -g to consider gravity)
%  - f_n1,tau_n1: force and torque vectors applied at the end effector, 0 if not in contact with environment
%  - Ai: 4x4xn matrix with the 4x4 DH homogeneous matrices
%  - dq, ddq: joint velocity and acceleration
%  - v: velocity multiplying matrix C(q,dq)
%  - m: n-dimensional array with link masses
%  - I: 3x3xn matrix containing inertia matrices
%  - rc: 3x1xn matrix with CoM vectors of link i expressed in frame i

n=size(Ai,3);

R=zeros(3,3,n);
for i=1:n
    R(:,:,i)=Ai(1:3,1:3,i);
end

w=zeros(3,1,n); 
w(:,:,1)=R(:,:,1)'*(w_0+[0;0;dq(1)]);

wa=zeros(3,1,n);
wa_0=zeros(3,1);
wa(:,:,1)=R(:,:,1)'*(wa_0+[0;0;v(1)]);

dw=zeros(3,1,n); 
dw(:,:,1)=R(:,:,1)'*(dw_0+[0;0;ddq(1)] + dq(1)*cross(wa_0,[0;0;1]));

a=zeros(3,1,n);
a(:,:,1)=R(:,:,1)'*a_0 + cross(dw(:,:,1),R(:,:,1)'*Ai(1:3,4,1)) + cross(w(:,:,1),cross(wa(:,:,1),R(:,:,1)'*Ai(1:3,4,1)));

ac=zeros(3,1,n);
ac(:,:,1)= a(:,:,1) + cross(dw(:,:,1),rc(:,:,1)) + cross(w(:,:,1),cross(wa(:,:,1),rc(:,:,1)));

%forward recursion
for i=2:n
    w(:,:,i)=R(:,:,i)'*(w(:,:,i-1)+[0;0;dq(i)]);
    wa(:,:,i)=R(:,:,i)'*(wa(:,:,i-1)+[0;0;v(i)]);
    dw(:,:,i)=R(:,:,i)'*( dw(:,:,i-1)+[0;0;ddq(i)] + dq(i)*(Smtrx(wa(:,:,i-1))*[0;0;1]));
    a(:,:,i)=R(:,:,i)'*a(:,:,i-1) + cross(dw(:,:,i),R(:,:,i)'*Ai(1:3,4,i)) + cross(w(:,:,i),cross(wa(:,:,i), R(:,:,i)'*Ai(1:3,4,i)));
    ac(:,:,i)= a(:,:,i) + cross(dw(:,:,i),rc(:,:,i)) + cross(w(:,:,i),cross(wa(:,:,i),rc(:,:,i)));
end

%backward recursion
f=zeros(3,1,n);
f(:,:,n)= f_n1 + m(n)*ac(:,:,n);
tau=zeros(3,1,n);
tau(:,:,n)= tau_n1 + cross(f_n1,rc(:,:,n)) - cross(f(:,:,n),R(:,:,n)'*Ai(1:3,4,n) + rc(:,:,n)) + I(:,:,n)*dw(:,:,n) + cross(wa(:,:,n),I(:,:,n)*w(:,:,n));
for i=n-1:-1:1
    f(:,:,i)= R(:,:,i+1)*f(:,:,i+1) + m(i)*ac(:,:,i);
    tau(:,:,i)= R(:,:,i+1)*tau(:,:,i+1) + cross(R(:,:,i+1)*f(:,:,i+1),rc(:,:,i)) - cross(f(:,:,i),R(:,:,i)'*Ai(1:3,4,i) + rc(:,:,i)) + I(:,:,i)*dw(:,:,i) + cross(wa(:,:,i),I(:,:,i)*w(:,:,i));
end

% projection
u=zeros(n,1);
for i=1:n
    u(i)=tau(:,:,i)'*R(3,:,i)';
end

== matlab function simulation/estimate velocity/reduced order observer: gain scheduling/MATLAB Function ==
  data: table input; A output
function A = DHMatrix(table)
% inputs:
%  -table: the DH parameters table, a n-vector of vectors composed with 
%  this structure: [alpha a d theta]
% output:
%  -A: cell array with homogeneous relative transformations from RF i-1 to
%   RF i
    nums = size(table);
    
    A = zeros(4,4,nums(1));
    
    for i = 1:nums(1)
        line = table(i, :);
        R = [cos(line(4)) -cos(line(1))*sin(line(4)) sin(line(1))*sin(line(4)) line(2)*cos(line(4));
             sin(line(4)) cos(line(1))*cos(line(4)) -sin(line(1))*cos(line(4)) line(2)*sin(line(4));
             0 sin(line(1)) cos(line(1)) line(3);
             0 0 0 1;];
        A(:,:,i) = R;
    end
   
end

== matlab function simulation/estimate velocity/reduced order observer: gain scheduling/MATLAB Function1 ==
  data: c0_bar input; eta input; r input; vbar input; lambda_1 input; kr output
function kr = gain_schedule(c0_bar,eta,r,vbar,lambda_1)
% return the continuous time dynamics given state  and input

kr = c0_bar*(eta+r*vbar)/(2*lambda_1);
end

== matlab function simulation/estimate velocity/reduced order observer: gain scheduling/MATLAB Function2 ==
  data: g input; Ai input; x2hat input; m input; I input; rc input; dz output; u input; k0 input; M output
function [dz,M] = obs_dynamics(g,Ai,x2hat,m,I,rc,u,k0)
% return the continuous time dynamics given state  and input

Cg = mod_newton_euler(zeros(3,1),zeros(3,1),g,zeros(3,1),zeros(3,1), ...
    Ai,x2hat,x2hat,zeros(3,1),m,I,rc);

M = zeros(3,3);
M(:,1) = mod_newton_euler(zeros(3,1),zeros(3,1),zeros(3,1),zeros(3,1),zeros(3,1), ...
        Ai,zeros(3,1),zeros(3,1),[1;0;0],m,I,rc);
M(:,2) = mod_newton_euler(zeros(3,1),zeros(3,1),zeros(3,1),zeros(3,1),zeros(3,1), ...
        Ai,zeros(3,1),zeros(3,1),[0;1;0],m,I,rc);
M(:,3) = mod_newton_euler(zeros(3,1),zeros(3,1),zeros(3,1),zeros(3,1),zeros(3,1), ...
        Ai,zeros(3,1),zeros(3,1),[0;0;1],m,I,rc);

dz = inv(M)*(-Cg+u)-k0*x2hat;
end

== matlab function simulation/estimate velocity/reduced order observer: gain scheduling/MATLAB Function3 ==
  data: x2hat input; vbar input; eta input; r input; r_new output
function r_new = r_dynamics(x2hat,vbar,eta,r)

mod = norm(x2hat);
gap_width = 2*eta;

if mod >= r*vbar-eta
    r_new=r+1;
elseif mod <= (r-1)*vbar+eta
    if mod >= (r-1)*vbar+eta-gap_width
        r_new=r;
    else
        r_new=r-1;
    end
else
    r_new=r;
end
r_new=max(r_new,1);
end

== matlab function simulation/estimate velocity/reduced order observer: gain scheduling/MATLAB Function4 ==
  data: x input; y output
function y = vector_norm(x)
y=norm(x);
end

== matlab function simulation/desired joint trajectory generator/generate dq,ddq ==
  data: q input size=[3,1]; v input size=[6,1]; dq output; a input size=[6,1]; ddq output
function [dq,ddq] = diff_inv_kin(q, v, a)
v=v(4:6);
a=a(4:6);
J = [-(sin(q(1))*(4*cos(q(2) + q(3)) + 5*cos(q(2))))/10, -(cos(q(1))*(4*sin(q(2) + q(3)) + 5*sin(q(2))))/10, -(2*sin(q(2) + q(3))*cos(q(1)))/5;
    (cos(q(1))*(4*cos(q(2) + q(3)) + 5*cos(q(2))))/10, -(sin(q(1))*(4*sin(q(2) + q(3)) + 5*sin(q(2))))/10, -(2*sin(q(2) + q(3))*sin(q(1)))/5;
                                            0,             (2*cos(q(2) + q(3)))/5 + cos(q(2))/2,          (2*cos(q(2) + q(3)))/5];
Jpinv=pinv(J);
dq = Jpinv*v;

Jdot = [  (2*dq(3)*sin(q(2) + q(3))*sin(q(1)))/5 - (dq(1)*cos(q(1))*(4*cos(q(2) + q(3)) + 5*cos(q(2))))/10 + (dq(2)*sin(q(1))*(4*sin(q(2) + q(3)) + 5*sin(q(2))))/10,   (dq(1)*sin(q(1))*(4*sin(q(2) + q(3)) + 5*sin(q(2))))/10 - (2*dq(3)*cos(q(2) + q(3))*cos(q(1)))/5 - (dq(2)*cos(q(1))*(4*cos(q(2) + q(3)) + 5*cos(q(2))))/10,   (2*dq(1)*sin(q(2) + q(3))*sin(q(1)))/5 - (2*dq(3)*cos(q(2) + q(3))*cos(q(1)))/5 - (2*dq(2)*cos(q(2) + q(3))*cos(q(1)))/5;
       - (dq(1)*sin(q(1))*(4*cos(q(2) + q(3)) + 5*cos(q(2))))/10 - (2*dq(3)*sin(q(2) + q(3))*cos(q(1)))/5 - (dq(2)*cos(q(1))*(4*sin(q(2) + q(3)) + 5*sin(q(2))))/10, - (dq(2)*sin(q(1))*(4*cos(q(2) + q(3)) + 5*cos(q(2))))/10 - (2*dq(3)*cos(q(2) + q(3))*sin(q(1)))/5 - (dq(1)*cos(q(1))*(4*sin(q(2) + q(3)) + 5*sin(q(2))))/10, - (2*dq(1)*sin(q(2) + q(3))*cos(q(1)))/5 - (2*dq(2)*cos(q(2) + q(3))*sin(q(1)))/5 - (2*dq(3)*cos(q(2) + q(3))*sin(q(1)))/5;
                                                                                                                                      0,                                                                  - (2*dq(3)*sin(q(2) + q(3)))/5 - dq(2)*((2*sin(q(2) + q(3)))/5 + sin(q(2))/2),                                                                    -(2*sin(q(2) + q(3))*(dq(2) + dq(3)))/5];
ddq = Jpinv*(a-Jdot*dq);

== matlab function simulation/desired joint trajectory generator/perform inverse kinematics ==
  data: p input size=[3,1]; q output
function q = inv_kin(p)
q = [0,0,0]';
L1=0.5; % link lengths [m]  
L2=0.5;
L3=0.4;
c3 = (p(1)^2+p(2)^2+(p(3)-L1)^2-L2^2-L3^2)/(2*L2*L3);

q(3)=-atan2(sqrt(1-c3^2),c3);

if p(1)^2+p(2)^2 >0
    q(1)=atan2(p(2),p(1));
end
if p(1)^2+p(2)^2+(p(3)-L1)^2 ~= 0
    sol=linsolve([L2+L3*cos(q(3)) -L3*sin(q(3)); L3*sin(q(3)) L2+L3*cos(q(3))], ...
            [cos(q(1))*p(1)+sin(q(1))*p(2);p(3)-L1]);
    q(2)=atan2(sol(2),sol(1));
end

== matlab function simulation/controller/MATLAB Function ==
  data: table input; A output
function A = DHMatrix(table)
% inputs:
%  -table: the DH parameters table, a n-vector of vectors composed with 
%  this structure: [alpha a d theta]
% output:
%  -A: cell array with homogeneous relative transformations from RF i-1 to
%   RF i
    nums = size(table);
    
    A = zeros(4,4,nums(1));
    
    for i = 1:nums(1)
        line = table(i, :);
        R = [cos(line(4)) -cos(line(1))*sin(line(4)) sin(line(1))*sin(line(4)) line(2)*cos(line(4));
             sin(line(4)) cos(line(1))*cos(line(4)) -sin(line(1))*cos(line(4)) line(2)*sin(line(4));
             0 sin(line(1)) cos(line(1)) line(3);
             0 0 0 1;];
        A(:,:,i) = R;
    end
   
end

== matlab function simulation/manipulator dynamics/MATLAB Function2 ==
  data: g input; Ai input; dq input; m input; I input; rc input; dx output; u input
function dx = ct_dynamics(g,Ai,dq,m,I,rc,u)
% return the continuous time dynamics given state  and input

Cg = mod_newton_euler(zeros(3,1),zeros(3,1),g,zeros(3,1),zeros(3,1), ...
    Ai,dq,dq,zeros(3,1),m,I,rc);

M = zeros(3,3);
M(:,1) = mod_newton_euler(zeros(3,1),zeros(3,1),zeros(3,1),zeros(3,1),zeros(3,1), ...
        Ai,zeros(3,1),zeros(3,1),[1;0;0],m,I,rc);
M(:,2) = mod_newton_euler(zeros(3,1),zeros(3,1),zeros(3,1),zeros(3,1),zeros(3,1), ...
        Ai,zeros(3,1),zeros(3,1),[0;1;0],m,I,rc);
M(:,3) = mod_newton_euler(zeros(3,1),zeros(3,1),zeros(3,1),zeros(3,1),zeros(3,1), ...
        Ai,zeros(3,1),zeros(3,1),[0;0;1],m,I,rc);

dx=[dq;
    inv(M)*(-Cg+u)];
end

== matlab function simulation/compute energy residual/MATLAB Function ==
  data: table input; A output
function A = DHMatrix(table)
% inputs:
%  -table: the DH parameters table, a n-vector of vectors composed with 
%  this structure: [alpha a d theta]
% output:
%  -A: cell array with homogeneous relative transformations from RF i-1 to
%   RF i
    nums = size(table);
    
    A = zeros(4,4,nums(1));
    
    for i = 1:nums(1)
        line = table(i, :);
        R = [cos(line(4)) -cos(line(1))*sin(line(4)) sin(line(1))*sin(line(4)) line(2)*cos(line(4));
             sin(line(4)) cos(line(1))*cos(line(4)) -sin(line(1))*cos(line(4)) line(2)*sin(line(4));
             0 sin(line(1)) cos(line(1)) line(3);
             0 0 0 1;];
        A(:,:,i) = R;
    end
   
end

== matlab function simulation/compute energy residual/MATLAB Function1 ==
  data: w_0 input; u output; dw_0 input; a_0 input; f_n1 input; tau_n1 input; Ai input; dq input; v input; ddq input; m input; I input; rc input
function u=mod_newton_euler(w_0,dw_0,a_0,f_n1,tau_n1,Ai,dq,v,ddq,m,I,rc)
% NE algorithm for robot dynamics with revolute joints
% inputs:
% - w_0, dw_0: angular velocity and acceleration of the base
%  - a_0: acceleration of the base (set this to -g to consider gravity)
%  - f_n1,tau_n1: force and torque vectors applied at the end effector, 0 if not in contact with environment
%  - Ai: 4x4xn matrix with the 4x4 DH homogeneous matrices
%  - dq, ddq: joint velocity and acceleration
%  - v: velocity multiplying matrix C(q,dq)
%  - m: n-dimensional array with link masses
%  - I: 3x3xn matrix containing inertia matrices
%  - rc: 3x1xn matrix with CoM vectors of link i expressed in frame i

n=size(Ai,3);

R=zeros(3,3,n);
for i=1:n
    R(:,:,i)=Ai(1:3,1:3,i);
end

w=zeros(3,1,n); 
w(:,:,1)=R(:,:,1)'*(w_0+[0;0;dq(1)]);

wa=zeros(3,1,n);
wa_0=zeros(3,1);
wa(:,:,1)=R(:,:,1)'*(wa_0+[0;0;v(1)]);

dw=zeros(3,1,n); 
dw(:,:,1)=R(:,:,1)'*(dw_0+[0;0;ddq(1)] + dq(1)*cross(wa_0,[0;0;1]));

a=zeros(3,1,n);
a(:,:,1)=R(:,:,1)'*a_0 + cross(dw(:,:,1),R(:,:,1)'*Ai(1:3,4,1)) + cross(w(:,:,1),cross(wa(:,:,1),R(:,:,1)'*Ai(1:3,4,1)));

ac=zeros(3,1,n);
ac(:,:,1)= a(:,:,1) + cross(dw(:,:,1),rc(:,:,1)) + cross(w(:,:,1),cross(wa(:,:,1),rc(:,:,1)));

%forward recursion
for i=2:n
    w(:,:,i)=R(:,:,i)'*(w(:,:,i-1)+[0;0;dq(i)]);
    wa(:,:,i)=R(:,:,i)'*(wa(:,:,i-1)+[0;0;v(i)]);
    dw(:,:,i)=R(:,:,i)'*( dw(:,:,i-1)+[0;0;ddq(i)] + dq(i)*(Smtrx(wa(:,:,i-1))*[0;0;1]));
    a(:,:,i)=R(:,:,i)'*a(:,:,i-1) + cross(dw(:,:,i),R(:,:,i)'*Ai(1:3,4,i)) + cross(w(:,:,i),cross(wa(:,:,i), R(:,:,i)'*Ai(1:3,4,i)));
    ac(:,:,i)= a(:,:,i) + cross(dw(:,:,i),rc(:,:,i)) + cross(w(:,:,i),cross(wa(:,:,i),rc(:,:,i)));
end

%backward recursion
f=zeros(3,1,n);
f(:,:,n)= f_n1 + m(n)*ac(:,:,n);
tau=zeros(3,1,n);
tau(:,:,n)= tau_n1 + cross(f_n1,rc(:,:,n)) - cross(f(:,:,n),R(:,:,n)'*Ai(1:3,4,n) + rc(:,:,n)) + I(:,:,n)*dw(:,:,n) + cross(wa(:,:,n),I(:,:,n)*w(:,:,n));
for i=n-1:-1:1
    f(:,:,i)= R(:,:,i+1)*f(:,:,i+1) + m(i)*ac(:,:,i);
    tau(:,:,i)= R(:,:,i+1)*tau(:,:,i+1) + cross(R(:,:,i+1)*f(:,:,i+1),rc(:,:,i)) - cross(f(:,:,i),R(:,:,i)'*Ai(1:3,4,i) + rc(:,:,i)) + I(:,:,i)*dw(:,:,i) + cross(wa(:,:,i),I(:,:,i)*w(:,:,i));
end

% projection
u=zeros(n,1);
for i=1:n
    u(i)=tau(:,:,i)'*R(3,:,i)';
end

== matlab function simulation/compute energy residual/MATLAB Function2 ==
  data: w_0 input; u output; dw_0 input; a_0 input; f_n1 input; tau_n1 input; Ai input; dq input; v input; ddq input; m input; I input; rc input
function u=mod_newton_euler(w_0,dw_0,a_0,f_n1,tau_n1,Ai,dq,v,ddq,m,I,rc)
% NE algorithm for robot dynamics with revolute joints
% inputs:
% - w_0, dw_0: angular velocity and acceleration of the base
%  - a_0: acceleration of the base (set this to -g to consider gravity)
%  - f_n1,tau_n1: force and torque vectors applied at the end effector, 0 if not in contact with environment
%  - Ai: 4x4xn matrix with the 4x4 DH homogeneous matrices
%  - dq, ddq: joint velocity and acceleration
%  - v: velocity multiplying matrix C(q,dq)
%  - m: n-dimensional array with link masses
%  - I: 3x3xn matrix containing inertia matrices
%  - rc: 3x1xn matrix with CoM vectors of link i expressed in frame i

n=size(Ai,3);

R=zeros(3,3,n);
for i=1:n
    R(:,:,i)=Ai(1:3,1:3,i);
end

w=zeros(3,1,n); 
w(:,:,1)=R(:,:,1)'*(w_0+[0;0;dq(1)]);

wa=zeros(3,1,n);
wa_0=zeros(3,1);
wa(:,:,1)=R(:,:,1)'*(wa_0+[0;0;v(1)]);

dw=zeros(3,1,n); 
dw(:,:,1)=R(:,:,1)'*(dw_0+[0;0;ddq(1)] + dq(1)*cross(wa_0,[0;0;1]));

a=zeros(3,1,n);
a(:,:,1)=R(:,:,1)'*a_0 + cross(dw(:,:,1),R(:,:,1)'*Ai(1:3,4,1)) + cross(w(:,:,1),cross(wa(:,:,1),R(:,:,1)'*Ai(1:3,4,1)));

ac=zeros(3,1,n);
ac(:,:,1)= a(:,:,1) + cross(dw(:,:,1),rc(:,:,1)) + cross(w(:,:,1),cross(wa(:,:,1),rc(:,:,1)));

%forward recursion
for i=2:n
    w(:,:,i)=R(:,:,i)'*(w(:,:,i-1)+[0;0;dq(i)]);
    wa(:,:,i)=R(:,:,i)'*(wa(:,:,i-1)+[0;0;v(i)]);
    dw(:,:,i)=R(:,:,i)'*( dw(:,:,i-1)+[0;0;ddq(i)] + dq(i)*(Smtrx(wa(:,:,i-1))*[0;0;1]));
    a(:,:,i)=R(:,:,i)'*a(:,:,i-1) + cross(dw(:,:,i),R(:,:,i)'*Ai(1:3,4,i)) + cross(w(:,:,i),cross(wa(:,:,i), R(:,:,i)'*Ai(1:3,4,i)));
    ac(:,:,i)= a(:,:,i) + cross(dw(:,:,i),rc(:,:,i)) + cross(w(:,:,i),cross(wa(:,:,i),rc(:,:,i)));
end

%backward recursion
f=zeros(3,1,n);
f(:,:,n)= f_n1 + m(n)*ac(:,:,n);
tau=zeros(3,1,n);
tau(:,:,n)= tau_n1 + cross(f_n1,rc(:,:,n)) - cross(f(:,:,n),R(:,:,n)'*Ai(1:3,4,n) + rc(:,:,n)) + I(:,:,n)*dw(:,:,n) + cross(wa(:,:,n),I(:,:,n)*w(:,:,n));
for i=n-1:-1:1
    f(:,:,i)= R(:,:,i+1)*f(:,:,i+1) + m(i)*ac(:,:,i);
    tau(:,:,i)= R(:,:,i+1)*tau(:,:,i+1) + cross(R(:,:,i+1)*f(:,:,i+1),rc(:,:,i)) - cross(f(:,:,i),R(:,:,i)'*Ai(1:3,4,i) + rc(:,:,i)) + I(:,:,i)*dw(:,:,i) + cross(wa(:,:,i),I(:,:,i)*w(:,:,i));
end

% projection
u=zeros(n,1);
for i=1:n
    u(i)=tau(:,:,i)'*R(3,:,i)';
end

== matlab function simulation/manipulator dynamics/MATLAB Function ==
  data: table input; A output
function A = DHMatrix(table)
% inputs:
%  -table: the DH parameters table, a n-vector of vectors composed with 
%  this structure: [alpha a d theta]
% output:
%  -A: cell array with homogeneous relative transformations from RF i-1 to
%   RF i
    nums = size(table);
    
    A = zeros(4,4,nums(1));
    
    for i = 1:nums(1)
        line = table(i, :);
        R = [cos(line(4)) -cos(line(1))*sin(line(4)) sin(line(1))*sin(line(4)) line(2)*cos(line(4));
             sin(line(4)) cos(line(1))*cos(line(4)) -sin(line(1))*cos(line(4)) line(2)*sin(line(4));
             0 sin(line(1)) cos(line(1)) line(3);
             0 0 0 1;];
        A(:,:,i) = R;
    end
   
end
